simulink model "TwoLinkPlanarRobotHybridControl_gen2"  (Simulink 7.9)
settings: Solver=ode1  StartTime=0.0  StopTime=10.0  FixedStep=0.01  RelTol=1e-3
values from neighbouring files (symbols this model uses):
  m = [1 1]    [FurutaPendulum_Dynamics.m]    (also in Question_2.m = [m_1 m_2]; test_ForwardDynamics.m = [1 1 1]; test_TwoLinkPlanarRobotDynamics.m = [m1 m2]; test_TwoLinkPlanarRobotHybridControl.m = [m1 m2])
  N = 5    [createEllipsoid.m]
  s = tf('s')    [Current_loop_bode.m]    (also in Question_1.m = 15)
  X = cos(0:2*pi/n:2*pi)    [createCylinder.m]
  Y = sin(0:2*pi/n:2*pi)    [createCylinder.m]
undefined symbols (not defined in the file or in its folder): Z
libraries: sm_lib x13, nesl_utility x9, simulink x1
settings Model: Creator=leavesdown_admin  LastModifiedBy=leavesdown_admin
settings ConfigurationSet: Description=SimMechanics 2G

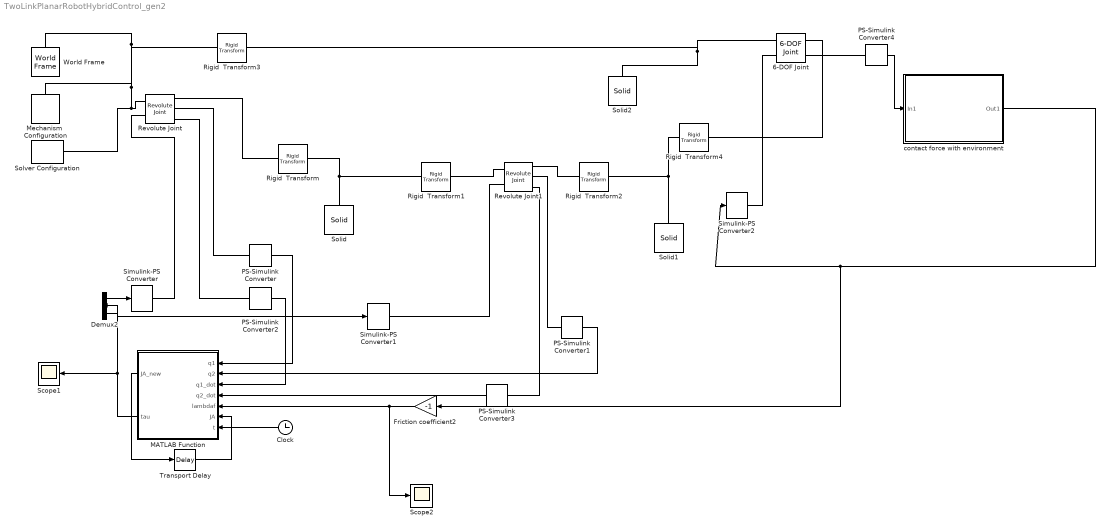
== system TwoLinkPlanarRobotHybridControl_gen2 ==
  6-DOF Joint : sm_lib/Joints/6-DOF Joint  SenseConstraintForceX=off  SenseConstraintForceY=off  SenseConstraintForceZ=off  SenseConstraintTorqueX=off  SenseConstraintTorqueY=off  SenseConstraintTorqueZ=off  ConstraintWrenchDir=FollowerOnBase  ConstraintWrenchFrame=BaseFrame  PxEquilibriumPosition=0  PxEquilibriumPositionUnits=m  PxSpringStiffness=0  PxSpringStiffnessUnits=N/m  PxDampingCoefficient=0  PxDampingCoefficientUnits=N/(m/s)  PxActuationMode=NoActuation  PxSensePosition=off  PxSenseVelocity=off  PxSenseAcceleration=off  PxSenseTorqueForce=off  PxPositionTargetValue=0  PxPositionTargetValueUnits=m  PxPositionTargetSpecify=off  PxPositionTargetPriority=High  PxVelocityTargetValue=0  PxVelocityTargetValueUnits=m/s  PxVelocityTargetSpecify=off  PxVelocityTargetPriority=High  PyEquilibriumPosition=0  PyEquilibriumPositionUnits=m  PySpringStiffness=0  PySpringStiffnessUnits=N/m  PyDampingCoefficient=0  PyDampingCoefficientUnits=N/(m/s)  PyActuationMode=TorqueForceActuation  PySensePosition=on  PySenseVelocity=off  PySenseAcceleration=off  PySenseTorqueForce=off  PyPositionTargetValue=0  PyPositionTargetValueUnits=m  PyPositionTargetSpecify=off  PyPositionTargetPriority=High  PyVelocityTargetValue=0  PyVelocityTargetValueUnits=m/s  PyVelocityTargetSpecify=off  PyVelocityTargetPriority=High  PzEquilibriumPosition=0  PzEquilibriumPositionUnits=m  PzSpringStiffness=0  PzSpringStiffnessUnits=N/m  PzDampingCoefficient=0  PzDampingCoefficientUnits=N/(m/s)  PzActuationMode=NoActuation  PzSensePosition=off  PzSenseVelocity=off  PzSenseAcceleration=off  PzSenseTorqueForce=off  PzPositionTargetValue=0  PzPositionTargetValueUnits=m  PzPositionTargetSpecify=off  PzPositionTargetPriority=High  PzVelocityTargetValue=0  PzVelocityTargetValueUnits=m/s  PzVelocityTargetSpecify=off  PzVelocityTargetPriority=High  SphDefPosRotationMethod=None  SphDefPosRotationAngleUnits=deg  SphDefPosRotationStandardAxis=+Z  SphDefPosRotationAngle=0  SphDefPosRotationArbitraryAxis=[0 0 1]  SphDefPosFollAlignAxisA=+X  SphDefPosBaseAlignAxisA=+Y  SphDefPosFollAlignAxisB=+Y  SphDefPosBaseAlignAxisB=+Z  SphEqPosRotationMethod=None  SphEqPosRotationAngleUnits=deg  SphEqPosRotationStandardAxis=+Z  SphEqPosRotationAngle=0  SphEqPosRotationArbitraryAxis=[0 0 1]  SphEqPosFollAlignAxisA=+X  SphEqPosBaseAlignAxisA=+Y  SphEqPosFollAlignAxisB=+Y  SphEqPosBaseAlignAxisB=+Z  SphSpringStiffness=0  SphSpringStiffnessUnits=N*m/deg  SphDampingCoefficient=0  SphDampingCoefficientUnits=N*m/(deg/s)  SphActuateTorqueX=off  SphActuateTorqueY=off  SphActuateTorqueZ=off  SphActuateTorque=off  SphActuationMode=NoActuation  SphActuationFrame=BaseFrame  SphSensePosition=off  SphSenseVelocityX=off  SphSenseVelocityY=off  SphSenseVelocityZ=off  SphSenseVelocity=off  SphSenseAccelerationX=off  SphSenseAccelerationY=off  SphSenseAccelerationZ=off  SphSenseAcceleration=off  SphSenseTorqueX=off  SphSenseTorqueY=off  SphSenseTorqueZ=off  SphSenseTorqueForce=off  SphSensingFrame=BaseFrame  SphPositionTargetRotationMethod=None  SphPositionTargetRotationAngleUnits=deg  SphPositionTargetRotationStandardAxis=+Z  SphPositionTargetRotationAngle=0  SphPositionTargetRotationArbitraryAxis=[0 0 1]  SphPositionTargetFollAlignAxisA=+X  SphPositionTargetBaseAlignAxisA=+Y  SphPositionTargetFollAlignAxisB=+Y  SphPositionTargetBaseAlignAxisB=+Z  SphPositionTargetSpecify=off  SphPositionTargetPriority=High  SphVelocityTargetValue=[0 0 0]  SphVelocityTargetValueUnits=deg/s  SphVelocityTargetSpecify=off  SphVelocityTargetPriority=High  SphVelocityTargetInFollowerFrame=on  BlockFunction=simmechanics.library.joints.sixdof_joint
  Clock : Clock
  Demux2 : Demux  Outputs=2
  Friction coefficient2 : Gain  Gain=-1
  MATLAB Function : MATLAB Function  TreatAsAtomicUnit=on
  Mechanism  Configuration : sm_lib/Utilities/Mechanism  Configuration  GravityVector=[0 -9.81 0]  GravityUnits=m/s^2  AllowGravitySignal=off  LinearizationDelta=0.001  BlockFunction=simmechanics.library.utilities.mechanism_configuration
  PS-Simulink Converter{,1..4} (5 alike) : nesl_utility/PS-Simulink Converter  PhysicalDomain=network_engine_domain  LeftPortType=input  RightPortType=output  SubClassName=ps_output  Unit=1  AffineConversion=off
  Revolute Joint : sm_lib/Joints/Revolute Joint  SenseConstraintForceX=off  SenseConstraintForceY=off  SenseConstraintForceZ=off  SenseConstraintTorqueX=off  SenseConstraintTorqueY=off  SenseConstraintTorqueZ=off  ConstraintWrenchDir=FollowerOnBase  ConstraintWrenchFrame=BaseFrame  EquilibriumPosition=0  EquilibriumPositionUnits=deg  SpringStiffness=0  SpringStiffnessUnits=N*m/deg  DampingCoefficient=50  DampingCoefficientUnits=N*m/(rad/s)  ActuationMode=TorqueForceActuation  SensePosition=on  SenseVelocity=on  SenseAcceleration=off  SenseTorqueForce=off  PositionTargetValue=0  PositionTargetValueUnits=rad  PositionTargetSpecify=on  PositionTargetPriority=High  VelocityTargetValue=0  VelocityTargetValueUnits=deg/s  VelocityTargetSpecify=off  VelocityTargetPriority=High  BlockFunction=simmechanics.library.joints.revolute_joint
  Revolute Joint1 : sm_lib/Joints/Revolute Joint  SenseConstraintForceX=off  SenseConstraintForceY=off  SenseConstraintForceZ=off  SenseConstraintTorqueX=off  SenseConstraintTorqueY=off  SenseConstraintTorqueZ=off  ConstraintWrenchDir=FollowerOnBase  ConstraintWrenchFrame=BaseFrame  EquilibriumPosition=0  EquilibriumPositionUnits=deg  SpringStiffness=0  SpringStiffnessUnits=N*m/deg  DampingCoefficient=50  DampingCoefficientUnits=N*m/(rad/s)  ActuationMode=TorqueForceActuation  SensePosition=on  SenseVelocity=on  SenseAcceleration=off  SenseTorqueForce=off  PositionTargetValue=pi/2  PositionTargetValueUnits=rad  PositionTargetSpecify=on  PositionTargetPriority=High  VelocityTargetValue=0  VelocityTargetValueUnits=deg/s  VelocityTargetSpecify=off  VelocityTargetPriority=High  BlockFunction=simmechanics.library.joints.revolute_joint
  Rigid  Transform{,1..2,4} (4 alike) : sm_lib/Frames and  Transforms/Rigid  Transform  TranslationMethod=Cartesian  TranslationLengthUnit=m  TranslationStandardAxis=+Z  TranslationStandardOffset=0  TranslationCartesianOffset=[0.5 0 0]  TranslationROffset=0  TranslationROffsetUnits=m  TranslationZOffset=0  TranslationZOffsetUnits=m  TranslationThetaOffset=0  TranslationThetaOffsetUnits=deg  RotationMethod=None  RotationAngleUnits=deg  RotationStandardAxis=+Z  RotationAngle=0  RotationArbitraryAxis=[0 0 1]  FollAlignAxisA=+X  BaseAlignAxisA=+Y  FollAlignAxisB=+Y  BaseAlignAxisB=+Z  BlockFunction=simmechanics.library.frames_transforms.rigid_transform
  Rigid  Transform3 : sm_lib/Frames and  Transforms/Rigid  Transform  TranslationMethod=Cartesian  TranslationLengthUnit=m  TranslationStandardAxis=+Z  TranslationStandardOffset=0  TranslationCartesianOffset=[1 1 0]  TranslationROffset=0  TranslationROffsetUnits=m  TranslationZOffset=0  TranslationZOffsetUnits=m  TranslationThetaOffset=0  TranslationThetaOffsetUnits=deg  RotationMethod=StandardAxis  RotationAngleUnits=rad  RotationStandardAxis=+Z  RotationAngle=-pi/4  RotationArbitraryAxis=[0 0 1]  FollAlignAxisA=+X  BaseAlignAxisA=+Y  FollAlignAxisB=+Y  BaseAlignAxisB=+Z  BlockFunction=simmechanics.library.frames_transforms.rigid_transform
  Scope1 : Scope
  Scope2 : Scope
      settings: YMin=0  YMax=20  SaveName=ScopeData3
  Simulink-PS Converter : nesl_utility/Simulink-PS Converter  PhysicalDomain=network_engine_domain  LeftPortType=input  RightPortType=output  SubClassName=ps_input  Unit=1  AffineConversion=off  InputFilterTimeConstant=.001  UdotUserProvided=[]  SimscapeFilterOrder=1  InputFiltering=off
  Simulink-PS Converter1 : nesl_utility/Simulink-PS Converter  PhysicalDomain=network_engine_domain  LeftPortType=input  RightPortType=output  SubClassName=ps_input  Unit=1  AffineConversion=off  InputFilterTimeConstant=.001  UdotUserProvided=[]  SimscapeFilterOrder=1  InputFiltering=off
  Simulink-PS Converter2 : nesl_utility/Simulink-PS Converter  PhysicalDomain=network_engine_domain  LeftPortType=input  RightPortType=output  SubClassName=ps_input  Unit=1  AffineConversion=off  InputFilterTimeConstant=.001  UdotUserProvided=[]  SimscapeFilterOrder=1  InputFiltering=off
  Solid : sm_lib/Body Elements/Solid  InertiaType=Custom  Mass=50  MassUnits=kg  CenterOfMass=[0 0 0]  CenterOfMassUnits=m  MomentsOfInertia=[0 10 10]  MomentsOfInertiaUnits=kg*m^2  ProductsOfInertia=[0 0 0]  ProductsOfInertiaUnits=kg*m^2  DensityBased=on  Density=1000  DensityUnits=kg/(m^3)  GraphicType=FromGeometry  MarkerShape=Sphere  MarkerSize=10  MarkerSizeUnits=m  GraphicVisPropType=SimpleVisualProperties  GraphicDiffuseColor=[0.5 0.5 0.5]  GraphicSpecularColor=[0.5 0.5 0.5 1.0]  GraphicAmbientColor=[0.15 0.15 0.15 1.0]  GraphicEmissiveColor=[0.0 0.0 0.0 1.0]  GraphicShininess=75  GraphicOpacity=1.0  GeometryShape=Brick  RectangleSize=[1 1]  RectangleSizeUnits=m  BrickDimensions=[1 0.1 0.1]  BrickDimensionUnits=m  CylinderRadius=0.1  CylinderRadiusUnits=m  CylinderLength=1  CylinderLengthUnits=m  SphereRadius=1  SphereRadiusUnits=m  EllipsoidRadii=[1 1 1]  EllipsoidRadiiUnits=m  ExtrusionCrossSection=[1 1; -1 1; -1 -1; 1 -1]  ExtrusionCrossSectionUnits=m  ExtrusionLength=1  ExtrusionLengthUnits=m  PolygonNumSides=3  PolygonOuterRadius=1  PolygonOuterRadiusUnits=m  ExtGeomFileUnits=m  BlockFunction=simmechanics.library.body_elements.solid
  Solid1 : sm_lib/Body Elements/Solid  InertiaType=Custom  Mass=50  MassUnits=kg  CenterOfMass=[0 0 0]  CenterOfMassUnits=m  MomentsOfInertia=[0 10 10]  MomentsOfInertiaUnits=kg*m^2  ProductsOfInertia=[0 0 0]  ProductsOfInertiaUnits=kg*m^2  DensityBased=on  Density=1000  DensityUnits=kg/(m^3)  GraphicType=FromGeometry  MarkerShape=Sphere  MarkerSize=10  MarkerSizeUnits=m  GraphicVisPropType=SimpleVisualProperties  GraphicDiffuseColor=[0.5 0.5 0.5]  GraphicSpecularColor=[0.5 0.5 0.5 1.0]  GraphicAmbientColor=[0.15 0.15 0.15 1.0]  GraphicEmissiveColor=[0.0 0.0 0.0 1.0]  GraphicShininess=75  GraphicOpacity=1.0  GeometryShape=Brick  RectangleSize=[1 1]  RectangleSizeUnits=m  BrickDimensions=[1 0.1 0.1]  BrickDimensionUnits=m  CylinderRadius=0.1  CylinderRadiusUnits=m  CylinderLength=1  CylinderLengthUnits=m  SphereRadius=1  SphereRadiusUnits=m  EllipsoidRadii=[1 1 1]  EllipsoidRadiiUnits=m  ExtrusionCrossSection=[1 1; -1 1; -1 -1; 1 -1]  ExtrusionCrossSectionUnits=m  ExtrusionLength=1  ExtrusionLengthUnits=m  PolygonNumSides=3  PolygonOuterRadius=1  PolygonOuterRadiusUnits=m  ExtGeomFileUnits=m  BlockFunction=simmechanics.library.body_elements.solid
  Solid2 : sm_lib/Body Elements/Solid  InertiaType=Custom  Mass=50  MassUnits=kg  CenterOfMass=[0 0 0]  CenterOfMassUnits=m  MomentsOfInertia=[0 10 10]  MomentsOfInertiaUnits=kg*m^2  ProductsOfInertia=[0 0 0]  ProductsOfInertiaUnits=kg*m^2  DensityBased=on  Density=1000  DensityUnits=kg/(m^3)  GraphicType=FromGeometry  MarkerShape=Sphere  MarkerSize=10  MarkerSizeUnits=m  GraphicVisPropType=SimpleVisualProperties  GraphicDiffuseColor=[0.5 0.5 0.5]  GraphicSpecularColor=[0.5 0.5 0.5 1.0]  GraphicAmbientColor=[0.15 0.15 0.15 1.0]  GraphicEmissiveColor=[0.0 0.0 0.0 1.0]  GraphicShininess=75  GraphicOpacity=1.0  GeometryShape=Brick  RectangleSize=[1 1]  RectangleSizeUnits=m  BrickDimensions=[2 0.1 2]  BrickDimensionUnits=m  CylinderRadius=0.1  CylinderRadiusUnits=m  CylinderLength=1  CylinderLengthUnits=m  SphereRadius=1  SphereRadiusUnits=m  EllipsoidRadii=[1 1 1]  EllipsoidRadiiUnits=m  ExtrusionCrossSection=[1 1; -1 1; -1 -1; 1 -1]  ExtrusionCrossSectionUnits=m  ExtrusionLength=1  ExtrusionLengthUnits=m  PolygonNumSides=3  PolygonOuterRadius=1  PolygonOuterRadiusUnits=m  ExtGeomFileUnits=m  BlockFunction=simmechanics.library.body_elements.solid
  Solver Configuration : nesl_utility/Solver Configuration  PhysicalDomain=network_engine_domain  LeftPortType=input  RightPortType=generic  SubClassName=solver  UseCustomDae=off  DoDC=off  ResidualTolerance=1e-9  UseLocalSolver=off  LocalSolverChoice=NE_BACKWARD_EULER_ADVANCER  LocalSolverSampleTime=.01  DoFixedCost=off  MaxNonlinIter=3  MaxModeIter=2  LinearAlgebra=Sparse  Accelerate=off  Profile=off  UseLocalSampling=off  DelaysMemoryBudget=1024
  Transport Delay : TransportDelay  DelayTime=0.01
  World Frame : sm_lib/Frames and  Transforms/World Frame  BlockFunction=simmechanics.library.frames_transforms.world_frame
  contact force with environment : Subsystem
  wires:
  PS-Simulink Converter/1 -> MATLAB Function/1(q1)
  MATLAB Function/2(tau) -> Demux2/1, Scope1/1
  Demux2/1 -> Simulink-PS Converter/1
  PS-Simulink Converter1/1 -> MATLAB Function/2(q2)
  Clock/1 -> MATLAB Function/7(t)
  Demux2/2 -> Simulink-PS Converter1/1
  MATLAB Function/1(JA_new) -> Transport Delay/1
  Transport Delay/1 -> MATLAB Function/6(JA)
  PS-Simulink Converter2/1 -> MATLAB Function/3(q1_dot)
  PS-Simulink Converter3/1 -> MATLAB Function/4(q2_dot)
  Friction coefficient2/1 -> MATLAB Function/5(lambdaf), Scope2/1
  PS-Simulink Converter4/1 -> contact force with environment/1(In1)
  contact force with environment/1(Out1) -> Simulink-PS Converter2/1, Friction coefficient2/1
  connections:
  World Frame/RConn1 -- Revolute Joint/LConn1 -- Solver Configuration/RConn1 -- Mechanism  Configuration/RConn1 -- Rigid  Transform3/LConn1
  Rigid  Transform/RConn1 -- Solid/RConn1 -- Rigid  Transform1/LConn1
  Rigid  Transform/LConn1 -- Revolute Joint/RConn1
  Rigid  Transform1/RConn1 -- Revolute Joint1/LConn1
  Revolute Joint1/RConn1 -- Rigid  Transform2/LConn1
  Rigid  Transform2/RConn1 -- Solid1/RConn1 -- Rigid  Transform4/LConn1
  Revolute Joint/RConn2 -- PS-Simulink Converter/LConn1
  Simulink-PS Converter/RConn1 -- Revolute Joint/LConn2
  Revolute Joint1/RConn2 -- PS-Simulink Converter1/LConn1
  Revolute Joint/RConn3 -- PS-Simulink Converter2/LConn1
  PS-Simulink Converter3/LConn1 -- Revolute Joint1/RConn3
  Simulink-PS Converter1/RConn1 -- Revolute Joint1/LConn2
  Rigid  Transform3/RConn1 -- Solid2/RConn1 -- 6-DOF Joint/LConn1
  Rigid  Transform4/RConn1 -- 6-DOF Joint/RConn1
  6-DOF Joint/RConn2 -- PS-Simulink Converter4/LConn1
  Simulink-PS Converter2/RConn1 -- 6-DOF Joint/LConn2

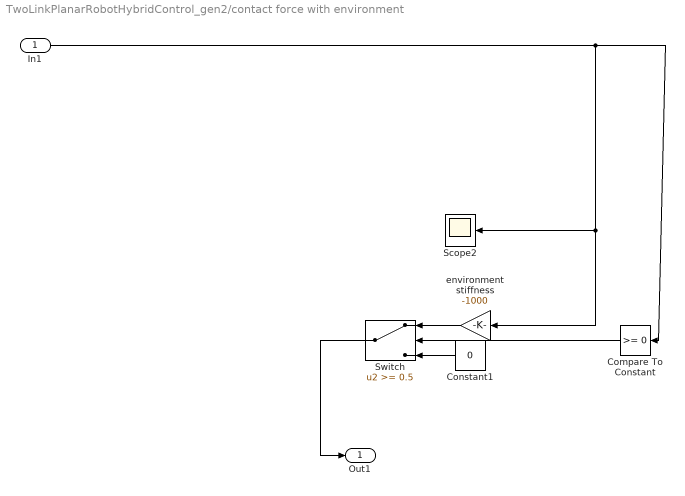
== system TwoLinkPlanarRobotHybridControl_gen2/contact force with environment ==
  In1 : Inport
  Compare To Constant : simulink/Logic and Bit Operations/Compare To Constant  relop=>=  const=0  OutDataTypeStr=uint8
  Constant1 : Constant  Value=0
  Scope2 : Scope
      settings: YMin=-0.85  YMax=-0.69  SaveName=ScopeData2
  Switch : Switch  Threshold=0.5
  environment stiffness : Gain  Gain=-1000
  Out1 : Outport
  wires:
  In1/1 -> Compare To Constant/1, environment stiffness/1, Scope2/1
  Compare To Constant/1 -> Switch/2
  environment stiffness/1 -> Switch/1
  Constant1/1 -> Switch/3
  Switch/1 -> Out1/1

== matlab function MATLAB Function ==
  data: JA_new output double; q1 input double; q2 input double; q1_dot input double; q2_dot input double; lambdaf input double; JA input double; tau output double; t input double
function [JA_new,tau]  = fcn(q1,q2,q1_dot,q2_dot,lambdaf,JA,t)
coder.extrinsic('Newton_Euler_Iteration');
coder.extrinsic('Jacobian');
coder.extrinsic('Forward_Kinematics');

q=[q1;q2];
q_dot=[q1_dot;q2_dot];
Jtype=[0;0];
    a1=1;a2=1;
    n=2;%number of joints
    m1=50;m2=50;
    m=[m1 m2]; %define mass constants
    Il1=10;Il2=10;
    I=zeros(3,3,2);
    I(:,:,1)=[0 0 0;0 Il1 0;0 0 Il1];I(:,:,2)=[0 0 0;0 Il2 0;0 0 Il2];%define inertia tensor
    l1=0.5;l2=0.5;
    r_C=[[l1-a1;0;0] [l2-a2;0;0]];%define com coordinates of each link
    kv=[50;50];%define viscous friction constants
    g=9.8;
    g0=[0;-g;0];%define gravity vector
    lambdafd=20;%desired contact force
    DH=[[0;q1;a1;0] [0;q2;a2;0]];
    B=zeros(2,2);
    for i=1:n
        q_ddot_temp=[0;0];
        q_ddot_temp(i)=1;
        B(:,i) = Newton_Euler_Iteration(DH, m, I, r_C, Jtype, [0;0], q_ddot_temp, [0;0;0]);
    end
    Coriolis_Gravity=zeros(2,1);
    Coriolis_Gravity=Newton_Euler_Iteration(DH, m, I, r_C, Jtype, q_dot, [0;0], g0);%compute C(q,\dot{q})\dot{q}+G(q)
    
    J=zeros(6,n);
    J=Jacobian(DH,Jtype);
    Sf=[cos(pi/4);sin(pi/4)];
    Sv=[-sin(pi/4);cos(pi/4)];
    JA_new=J(1:2,:);
    dt=0.01;
    JA_dot=(JA_new-JA)./dt;
    Bm=50;Dm=400;Km=10;
    A_lump=zeros(4,4,n);
    A_lump = Forward_Kinematics(DH);
    Ae=A_lump(:,:,n);
    temp=[Sf Sv]'*[Ae(1,4);Ae(2,4)];
    sf=temp(1);sv=temp(2);    
    temp=[Sf Sv]'*JA*q_dot;
    sf_dot=temp(1);sv_dot=temp(2);
    sfc=sqrt(2);
    lambdav=0;%friction force in unconstrained direction is zero
    
    %desired trajectory in unconstrained direction
    svd=0.5*sin(2*pi/2*t);
    svd_dot=0.5*2*pi/2*cos(2*pi/2*t);
    svd_ddot=-0.5*(2*pi/2)^2*sin(2*pi/2*t);
    
    %position control law in unconstrained direction
    ev=sv-svd;
    ev_dot=sv_dot-svd_dot;
    Kp=25;Kd=5;
    av=svd_ddot-Kp*ev-Kd*ev_dot;
    
    %direct force control in constrained direction
    k_hat=1000;%estimation of contact stiffness k
    %calculate the estimate of velocity in the constrained direction
    %(lambdaf_dot)
    if sf<sfc
        lambdaf_dot_hat=0;
    else
        lambdaf_dot_hat=k_hat*sf_dot;
    end
    kp=100;kd=20;
    af=-kp/k_hat*(lambdaf-lambdafd)-kd/k_hat*lambdaf_dot_hat;
    
    % impedance control in constrained direction
%     Mm=50;Dm=400;Km=10;
%     sfd=sfc+lambdafd/Km;
%     af=1/Mm*(-Dm*(sf_dot)-Km*(sf-sfd)-lambdaf);
    
    %total control law
    tau=Coriolis_Gravity+kv.*q_dot+JA'*(Sf*lambdaf+Sv*lambdav)+B*JA'*inv(JA*JA'+0.01.*eye(2))*(-JA_dot*q_dot+Sf*af+Sv*av);
